simulink model "sistemidentifikasi"  (Simulink 8.6)
settings: Solver=ode45  StartTime=0.0  StopTime=20  RelTol=1e-3
undefined symbols (not defined in the file or in its folder): denuma, denumd, numa, numd
settings Model: Creator=bHe  LastModifiedBy=wafiq
settings DebuggingCC: FcnCallInpInsideContextMsg=UseLocalSettings

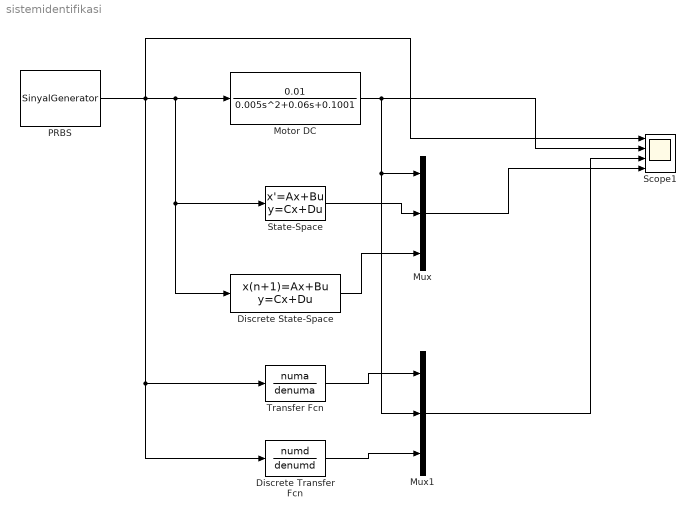
== system sistemidentifikasi ==
  Discrete Transfer Fcn : DiscreteTransferFcn  Numerator=numd  Denominator=denumd  InputProcessing=Columns as channels (frame based)  SampleTime=0.01  a0EqualsOne=on  RndMeth=Nearest
      settings: LockScale=on
  Discrete State-Space : DiscreteStateSpace  A="[0.9997   -0.01947   0.001716;   0.04475     0.8918    0.05751; -0.006716  -0.004705     0.9936]"  B=|  C="[ -0.8353  0.09902   -0.834]"  D=0  SampleTime=0.01
      | [0.002085; 0.01668
      | ; -0.0002232]
  Motor DC : TransferFcn  Numerator=[0.01]  Denominator=[0.005 0.06 0.1001]
  Mux : Mux  Inputs=3
  Mux1 : Mux  Inputs=3
  PRBS : FromWorkspace  VariableName=SinyalGenerator  SampleTime=0.01
  Scope1 : Scope  NumInputPorts=4
  State-Space : StateSpace  A="[0.01614    -2.06   0.2328; 4.756   -11.39      6.1;  -0.6622  -0.5065  -0.6299]"  B="[0.226; 1.76;  -0.01738]"  C="[ -0.8353  0.09902   -0.834]"  D=[0]  X0=0
  Transfer Fcn : TransferFcn  Numerator=numa  Denominator=denuma
  wires:
  Mux1/1 -> Scope1/3
  Transfer Fcn/1 -> Mux1/1
  Discrete Transfer Fcn/1 -> Mux1/3
  PRBS/1 -> Transfer Fcn/1, Discrete Transfer Fcn/1, Discrete State-Space/1, State-Space/1, Motor DC/1, Scope1/1
  Motor DC/1 -> Mux1/2, Mux/1, Scope1/2
  Mux/1 -> Scope1/4
  State-Space/1 -> Mux/2
  Discrete State-Space/1 -> Mux/3
